simulink library "calcDynamicPressure"  (R2020a)
settings: Solver=VariableStepAuto  StartTime=0.0  StopTime=10.0  RelTol=1e-3
settings Model: Creator=Ayaz  LastModifiedBy=Ayaz

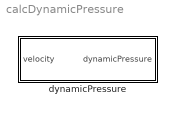
== system calcDynamicPressure ==
  dynamicPressure : Subsystem  mask{flowDensity=nan}
      mask prompts: flowDensity "Flow density [kg/m^3]"

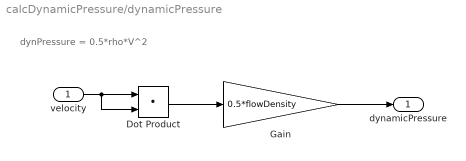
== system calcDynamicPressure/dynamicPressure ==
  note: dynPressure = 0.5*rho*V^2
  velocity : Inport
  Dot Product : DotProduct  InputSameDT=on  OutDataTypeStr=Inherit: Inherit via internal rule
  Gain : Gain  Gain=0.5*flowDensity
  dynamicPressure : Outport
  wires:
  velocity/1 -> Dot Product/2, Dot Product/1
  Dot Product/1 -> Gain/1
  Gain/1 -> dynamicPressure/1
